simulink model "Inverse_dynamic_Cartesian_aJacobian"  (R2020b)
settings: Solver=VariableStepAuto  StartTime=0.0  StopTime=10.0  RelTol=1e-3
(part 5 of 5)

== matlab function Inverse_dynamic_Cartesian_aJacobian/Controller/MATLAB Function ==
  data: Minimal input size=6; Minimald input; Jd output; Theta input size=6; Thetad input size=6
function Jd = JdAnalytical(Minimal,Minimald,Theta,Thetad)
alpha=Minimal(4);
beta=Minimal(5);
gamma=Minimal(6);
alphad=Minimald(4);
betad=Minimald(5);
gammad=Minimald(6);
t1=Theta(1);
t2=Theta(2);
t3=Theta(3);
t4=Theta(4);
t5=Theta(5);
t6=Theta(6);
td1=Thetad(1);
td2=Thetad(2);
td3=Thetad(3);
td4=Thetad(4);
td5=Thetad(5);
td6=Thetad(6);

Jd = [td2*(408*cos(t2)*sin(t1) - 376*sin(t1)*sin(t2)*sin(t3) + 376*cos(t2)*cos(t3)*sin(t1) + (205*cos(t2)*cos(t3)*cos(t4)*sin(t1))/2 - (205*cos(t2)*sin(t1)*sin(t3)*sin(t4))/2 - (205*cos(t3)*sin(t1)*sin(t2)*sin(t4))/2 - (205*cos(t4)*sin(t1)*sin(t2)*sin(t3))/2 + 94*cos(t2)*cos(t3)*sin(t1)*sin(t4)*sin(t5) + 94*cos(t2)*cos(t4)*sin(t1)*sin(t3)*sin(t5) + 94*cos(t3)*cos(t4)*sin(t1)*sin(t2)*sin(t5) - 94*sin(t1)*sin(t2)*sin(t3)*sin(t4)*sin(t5)) + td1*(408*cos(t1)*sin(t2) - (281*sin(t1))/2 - 94*cos(t5)*sin(t1) + 376*cos(t1)*cos(t2)*sin(t3) + 376*cos(t1)*cos(t3)*sin(t2) + (205*cos(t1)*cos(t2)*cos(t3)*sin(t4))/2 + (205*cos(t1)*cos(t2)*cos(t4)*sin(t3))/2 + (205*cos(t1)*cos(t3)*cos(t4)*sin(t2))/2 - (205*cos(t1)*sin(t2)*sin(t3)*sin(t4))/2 - 94*cos(t1)*cos(t2)*cos(t3)*cos(t4)*sin(t5) + 94*cos(t1)*cos(t2)*sin(t3)*sin(t4)*sin(t5) + 94*cos(t1)*cos(t3)*sin(t2)*sin(t4)*sin(t5) + 94*cos(t1)*cos(t4)*sin(t2)*sin(t3)*sin(t5)) + td4*((205*cos(t2)*cos(t3)*cos(t4)*sin(t1))/2 - (205*cos(t2)*sin(t1)*sin(t3)*sin(t4))/2 - (205*cos(t3)*sin(t1)*sin(t2)*sin(t4))/2 - (205*cos(t4)*sin(t1)*sin(t2)*sin(t3))/2 + 94*cos(t2)*cos(t3)*sin(t1)*sin(t4)*sin(t5) + 94*cos(t2)*cos(t4)*sin(t1)*sin(t3)*sin(t5) + 94*cos(t3)*cos(t4)*sin(t1)*sin(t2)*sin(t5) - 94*sin(t1)*sin(t2)*sin(t3)*sin(t4)*sin(t5)), td1*sin(t1)*((205*cos(t2 + t3 + t4))/2 - 47*cos(t2 + t3 + t4 + t5) + 376*cos(t2 + t3) + 408*cos(t2) + 47*cos(t2 + t3 + t4 - t5)) + td2*cos(t1)*(47*sin(t2 + t3 + t4 - t5) + (205*sin(t2 + t3 + t4))/2 - 47*sin(t2 + t3 + t4 + t5) + 376*sin(t2 + t3) + 408*sin(t2)) + td4*cos(t1)*(47*sin(t2 + t3 + t4 - t5) + (205*sin(t2 + t3 + t4))/2 - 47*sin(t2 + t3 + t4 + t5)), td2*cos(t1)*(47*sin(t2 + t3 + t4 - t5) + (205*sin(t2 + t3 + t4))/2 - 47*sin(t2 + t3 + t4 + t5) + 376*sin(t2 + t3)) + td1*sin(t1)*((205*cos(t2 + t3 + t4))/2 - 47*cos(t2 + t3 + t4 + t5) + 376*cos(t2 + t3) + 47*cos(t2 + t3 + t4 - t5)) + td4*cos(t1)*(47*sin(t2 + t3 + t4 - t5) + (205*sin(t2 + t3 + t4))/2 - 47*sin(t2 + t3 + t4 + t5)), td1*sin(t1)*((205*cos(t2 + t3 + t4))/2 - 47*cos(t2 + t3 + t4 + t5) + 47*cos(t2 + t3 + t4 - t5)) + td2*cos(t1)*(47*sin(t2 + t3 + t4 - t5) + (205*sin(t2 + t3 + t4))/2 - 47*sin(t2 + t3 + t4 + t5)) + td4*cos(t1)*(47*sin(t2 + t3 + t4 - t5) + (205*sin(t2 + t3 + t4))/2 - 47*sin(t2 + t3 + t4 + t5)),                                                                                                                                                                                                                                                                                                                                                                                                                                                                                                        94*td1*cos(t2)*cos(t5)*sin(t1)*sin(t3)*sin(t4) - 94*td2*sin(t2 + t3 + t4)*cos(t1)*cos(t5) - 94*td4*sin(t2 + t3 + t4)*cos(t1)*cos(t5) - 94*td1*cos(t2)*cos(t3)*cos(t4)*cos(t5)*sin(t1) - 94*td1*cos(t1)*sin(t5) + 94*td1*cos(t3)*cos(t5)*sin(t1)*sin(t2)*sin(t4) + 94*td1*cos(t4)*cos(t5)*sin(t1)*sin(t2)*sin(t3),                                                                                                                                                                                                                                                                                                                                                                                                                                                                                                                                                                                                                                                                                                                                                                                                                                                                                                                                                                                                                                                                                                                                                                                                                                                                                                                                             0
td1*((281*cos(t1))/2 + 94*cos(t1)*cos(t5) + 408*sin(t1)*sin(t2) + 376*cos(t2)*sin(t1)*sin(t3) + 376*cos(t3)*sin(t1)*sin(t2) + (205*cos(t2)*cos(t3)*sin(t1)*sin(t4))/2 + (205*cos(t2)*cos(t4)*sin(t1)*sin(t3))/2 + (205*cos(t3)*cos(t4)*sin(t1)*sin(t2))/2 - (205*sin(t1)*sin(t2)*sin(t3)*sin(t4))/2 - 94*cos(t2)*cos(t3)*cos(t4)*sin(t1)*sin(t5) + 94*cos(t2)*sin(t1)*sin(t3)*sin(t4)*sin(t5) + 94*cos(t3)*sin(t1)*sin(t2)*sin(t4)*sin(t5) + 94*cos(t4)*sin(t1)*sin(t2)*sin(t3)*sin(t5)) - td2*(408*cos(t1)*cos(t2) - 376*cos(t1)*sin(t2)*sin(t3) + 376*cos(t1)*cos(t2)*cos(t3) + (205*cos(t1)*cos(t2)*cos(t3)*cos(t4))/2 - (205*cos(t1)*cos(t2)*sin(t3)*sin(t4))/2 - (205*cos(t1)*cos(t3)*sin(t2)*sin(t4))/2 - (205*cos(t1)*cos(t4)*sin(t2)*sin(t3))/2 + 94*cos(t1)*cos(t2)*cos(t3)*sin(t4)*sin(t5) + 94*cos(t1)*cos(t2)*cos(t4)*sin(t3)*sin(t5) + 94*cos(t1)*cos(t3)*cos(t4)*sin(t2)*sin(t5) - 94*cos(t1)*sin(t2)*sin(t3)*sin(t4)*sin(t5)) - td4*((205*cos(t1)*cos(t2)*cos(t3)*cos(t4))/2 - (205*cos(t1)*cos(t2)*sin(t3)*sin(t4))/2 - (205*cos(t1)*cos(t3)*sin(t2)*sin(t4))/2 - (205*cos(t1)*cos(t4)*sin(t2)*sin(t3))/2 + 94*cos(t1)*cos(t2)*cos(t3)*sin(t4)*sin(t5) + 94*cos(t1)*cos(t2)*cos(t4)*sin(t3)*sin(t5) + 94*cos(t1)*cos(t3)*cos(t4)*sin(t2)*sin(t5) - 94*cos(t1)*sin(t2)*sin(t3)*sin(t4)*sin(t5)), td4*sin(t1)*(47*sin(t2 + t3 + t4 - t5) + (205*sin(t2 + t3 + t4))/2 - 47*sin(t2 + t3 + t4 + t5)) - td1*cos(t1)*((205*cos(t2 + t3 + t4))/2 - 47*cos(t2 + t3 + t4 + t5) + 376*cos(t2 + t3) + 408*cos(t2) + 47*cos(t2 + t3 + t4 - t5)) + td2*sin(t1)*(47*sin(t2 + t3 + t4 - t5) + (205*sin(t2 + t3 + t4))/2 - 47*sin(t2 + t3 + t4 + t5) + 376*sin(t2 + t3) + 408*sin(t2)), td4*sin(t1)*(47*sin(t2 + t3 + t4 - t5) + (205*sin(t2 + t3 + t4))/2 - 47*sin(t2 + t3 + t4 + t5)) + td2*sin(t1)*(47*sin(t2 + t3 + t4 - t5) + (205*sin(t2 + t3 + t4))/2 - 47*sin(t2 + t3 + t4 + t5) + 376*sin(t2 + t3)) - td1*cos(t1)*((205*cos(t2 + t3 + t4))/2 - 47*cos(t2 + t3 + t4 + t5) + 376*cos(t2 + t3) + 47*cos(t2 + t3 + t4 - t5)), td2*sin(t1)*(47*sin(t2 + t3 + t4 - t5) + (205*sin(t2 + t3 + t4))/2 - 47*sin(t2 + t3 + t4 + t5)) + td4*sin(t1)*(47*sin(t2 + t3 + t4 - t5) + (205*sin(t2 + t3 + t4))/2 - 47*sin(t2 + t3 + t4 + t5)) - td1*cos(t1)*((205*cos(t2 + t3 + t4))/2 - 47*cos(t2 + t3 + t4 + t5) + 47*cos(t2 + t3 + t4 - t5)),                                                                                                                                                                                                                                                                                                                                                                                                                                                                                                        94*td1*cos(t1)*cos(t2)*cos(t3)*cos(t4)*cos(t5) - 94*td2*sin(t2 + t3 + t4)*cos(t5)*sin(t1) - 94*td4*sin(t2 + t3 + t4)*cos(t5)*sin(t1) - 94*td1*sin(t1)*sin(t5) - 94*td1*cos(t1)*cos(t2)*cos(t5)*sin(t3)*sin(t4) - 94*td1*cos(t1)*cos(t3)*cos(t5)*sin(t2)*sin(t4) - 94*td1*cos(t1)*cos(t4)*cos(t5)*sin(t2)*sin(t3),                                                                                                                                                                                                                                                                                                                                                                                                                                                                                                                                                                                                                                                                                                                                                                                                                                                                                                                                                                                                                                                                                                                                                                                                                                                                                                                                             0
                                                                                                                                                                                                                                                                                                                                                                                                                                                                                                                                                                                                                                                                                                                                                                                                                                                                                                                                                                                                                                                                                                                                                                                                                                                                                                             0,                                                                                                                                                  - td2*((205*cos(t2 + t3 + t4))/2 - 47*cos(t2 + t3 + t4 + t5) + 376*cos(t2 + t3) + 408*cos(t2) + 47*cos(t2 + t3 + t4 - t5)) - td4*((205*cos(t2 + t3 + t4))/2 - 47*cos(t2 + t3 + t4 + t5) + 47*cos(t2 + t3 + t4 - t5)),                                                                                                                                    - td4*((205*cos(t2 + t3 + t4))/2 - 47*cos(t2 + t3 + t4 + t5) + 47*cos(t2 + t3 + t4 - t5)) - td2*((205*cos(t2 + t3 + t4))/2 - 47*cos(t2 + t3 + t4 + t5) + 376*cos(t2 + t3) + 47*cos(t2 + t3 + t4 - t5)),                                                                                                                                                                                                    -((td2 + td4)*(205*cos(t2 + t3 + t4) - 94*cos(t2 + t3 + t4 + t5) + 94*cos(t2 + t3 + t4 - t5)))/2,                                                                                                                                                                                                                                                                                                                                                                                                                                                                                                                                                                                                                                                                                                                                                        47*(td2 + td4)*(cos(t2 + t3 + t4 + t5) + cos(t2 + t3 + t4 - t5)),                                                                                                                                                                                                                                                                                                                                                                                                                                                                                                                                                                                                                                                                                                                                                                                                                                                                                                                                                                                                                                                                                                                                                                                                                                                                                                                                             0
                                                                                                                                                                                                                                                                                                                                                                                                                                                                                                                                                                                                                                                                                                                                                                                                                                                                                                                                                                                                                                                                                                                                                                                                                                                                                                             0,                                                                                         (cos(t1)*(betad*sin(alpha) - alphad*cos(alpha)*cos(beta)*sin(beta)))/(cos(beta)^2 - 1) - (sin(t1)*(betad*cos(alpha) + alphad*cos(beta)*sin(alpha)*sin(beta)))/(cos(beta)^2 - 1) - (td1*cos(alpha)*cos(beta)*cos(t1))/sin(beta) - (td1*cos(beta)*sin(alpha)*sin(t1))/sin(beta),                                                             (cos(t1)*(betad*sin(alpha) - alphad*cos(alpha)*cos(beta)*sin(beta)))/(cos(beta)^2 - 1) - (sin(t1)*(betad*cos(alpha) + alphad*cos(beta)*sin(alpha)*sin(beta)))/(cos(beta)^2 - 1) - (td1*cos(alpha)*cos(beta)*cos(t1))/sin(beta) - (td1*cos(beta)*sin(alpha)*sin(t1))/sin(beta),                       (cos(t1)*(betad*sin(alpha) - alphad*cos(alpha)*cos(beta)*sin(beta)))/(cos(beta)^2 - 1) - (sin(t1)*(betad*cos(alpha) + alphad*cos(beta)*sin(alpha)*sin(beta)))/(cos(beta)^2 - 1) - (td1*cos(alpha)*cos(beta)*cos(t1))/sin(beta) - (td1*cos(beta)*sin(alpha)*sin(t1))/sin(beta), (betad*(sin(alpha) + (cos(beta)^2*sin(alpha))/sin(beta)^2) - (alphad*cos(alpha)*cos(beta))/sin(beta))*(cos(t1 + t2 + t3 + t4)/2 - cos(t2 - t1 + t3 + t4)/2) - td4*sin(t2 + t3 + t4) - td2*sin(t2 + t3 + t4) - (betad*(cos(alpha) + (cos(alpha)*cos(beta)^2)/sin(beta)^2) + (alphad*cos(beta)*sin(alpha))/sin(beta))*(sin(t2 - t1 + t3 + t4)/2 + sin(t1 + t2 + t3 + t4)/2) - (cos(beta)*sin(alpha)*(td2*(sin(t2 - t1 + t3 + t4)/2 - sin(t1 + t2 + t3 + t4)/2) - td1*(sin(t2 - t1 + t3 + t4)/2 + sin(t1 + t2 + t3 + t4)/2) + td4*(sin(t2 - t1 + t3 + t4)/2 - sin(t1 + t2 + t3 + t4)/2)))/sin(beta) + (cos(alpha)*cos(beta)*(td1*(cos(t1 + t2 + t3 + t4)/2 - cos(t2 - t1 + t3 + t4)/2) + td2*(cos(t1 + t2 + t3 + t4)/2 + cos(t2 - t1 + t3 + t4)/2) + td4*(cos(t1 + t2 + t3 + t4)/2 + cos(t2 - t1 + t3 + t4)/2)))/sin(beta), ((betad*cos(alpha) + alphad*cos(beta)*sin(alpha)*sin(beta))*(cos(t1)*cos(t2)*sin(t3)*sin(t4)*sin(t5) - cos(t1)*cos(t2)*cos(t3)*cos(t4)*sin(t5) - cos(t5)*sin(t1) + cos(t1)*cos(t3)*sin(t2)*sin(t4)*sin(t5) + cos(t1)*cos(t4)*sin(t2)*sin(t3)*sin(t5)))/(cos(beta)^2 - 1) - (td4*(sin(t2 + t3 + t4 - t5) - sin(t2 + t3 + t4 + t5)))/2 - (td2*(sin(t2 + t3 + t4 - t5) - sin(t2 + t3 + t4 + t5)))/2 + ((betad*sin(alpha) - alphad*cos(alpha)*cos(beta)*sin(beta))*(cos(t1)*cos(t5) - cos(t2)*cos(t3)*cos(t4)*sin(t1)*sin(t5) + cos(t2)*sin(t1)*sin(t3)*sin(t4)*sin(t5) + cos(t3)*sin(t1)*sin(t2)*sin(t4)*sin(t5) + cos(t4)*sin(t1)*sin(t2)*sin(t3)*sin(t5)))/(cos(beta)^2 - 1) + (cos(beta)*sin(alpha)*(td2*sin(t2 + t3 + t4)*sin(t1)*sin(t5) - td1*cos(t5)*sin(t1) + td4*sin(t2 + t3 + t4)*sin(t1)*sin(t5) - td1*cos(t1)*cos(t2)*cos(t3)*cos(t4)*sin(t5) + td1*cos(t1)*cos(t2)*sin(t3)*sin(t4)*sin(t5) + td1*cos(t1)*cos(t3)*sin(t2)*sin(t4)*sin(t5) + td1*cos(t1)*cos(t4)*sin(t2)*sin(t3)*sin(t5)))/sin(beta) - (cos(alpha)*cos(beta)*(td1*cos(t1)*cos(t5) - td2*sin(t2 + t3 + t4)*cos(t1)*sin(t5) - td4*sin(t2 + t3 + t4)*cos(t1)*sin(t5) - td1*cos(t2)*cos(t3)*cos(t4)*sin(t1)*sin(t5) + td1*cos(t2)*sin(t1)*sin(t3)*sin(t4)*sin(t5) + td1*cos(t3)*sin(t1)*sin(t2)*sin(t4)*sin(t5) + td1*cos(t4)*sin(t1)*sin(t2)*sin(t3)*sin(t5)))/sin(beta)
                                                                                                                                                                                                                                                                                                                                                                                                                                                                                                                                                                                                                                                                                                                                                                                                                                                                                                                                                                                                                                                                                                                                                                                                                                                                                                             0,                                                                                                                                                                                                                                                                                                                                        sin(alpha - t1)*(alphad - td1),                                                                                                                                                                                                                                                                                                            sin(alpha - t1)*(alphad - td1),                                                                                                                                                                                                                                                                      sin(alpha - t1)*(alphad - td1),                                                                                                                                                                                                                                                                                                                                                                                                                                                                             (alphad*sin(alpha - t1 + t2 + t3 + t4))/2 + (alphad*sin(t1 - alpha + t2 + t3 + t4))/2 - (td1*sin(alpha - t1 + t2 + t3 + t4))/2 - (td1*sin(t1 - alpha + t2 + t3 + t4))/2 + (td2*sin(alpha - t1 + t2 + t3 + t4))/2 - (td2*sin(t1 - alpha + t2 + t3 + t4))/2 + (td4*sin(alpha - t1 + t2 + t3 + t4))/2 - (td4*sin(t1 - alpha + t2 + t3 + t4))/2,                                                                                                                                                                                                                                                                                               alphad*sin(alpha)*(cos(t1)*cos(t5) - cos(t2)*cos(t3)*cos(t4)*sin(t1)*sin(t5) + cos(t2)*sin(t1)*sin(t3)*sin(t4)*sin(t5) + cos(t3)*sin(t1)*sin(t2)*sin(t4)*sin(t5) + cos(t4)*sin(t1)*sin(t2)*sin(t3)*sin(t5)) - sin(alpha)*(td1*cos(t1)*cos(t5) - td2*sin(t2 + t3 + t4)*cos(t1)*sin(t5) - td4*sin(t2 + t3 + t4)*cos(t1)*sin(t5) - td1*cos(t2)*cos(t3)*cos(t4)*sin(t1)*sin(t5) + td1*cos(t2)*sin(t1)*sin(t3)*sin(t4)*sin(t5) + td1*cos(t3)*sin(t1)*sin(t2)*sin(t4)*sin(t5) + td1*cos(t4)*sin(t1)*sin(t2)*sin(t3)*sin(t5)) - cos(alpha)*(td2*sin(t2 + t3 + t4)*sin(t1)*sin(t5) - td1*cos(t5)*sin(t1) + td4*sin(t2 + t3 + t4)*sin(t1)*sin(t5) - td1*cos(t1)*cos(t2)*cos(t3)*cos(t4)*sin(t5) + td1*cos(t1)*cos(t2)*sin(t3)*sin(t4)*sin(t5) + td1*cos(t1)*cos(t3)*sin(t2)*sin(t4)*sin(t5) + td1*cos(t1)*cos(t4)*sin(t2)*sin(t3)*sin(t5)) + alphad*cos(alpha)*(cos(t1)*cos(t2)*sin(t3)*sin(t4)*sin(t5) - cos(t1)*cos(t2)*cos(t3)*cos(t4)*sin(t5) - cos(t5)*sin(t1) + cos(t1)*cos(t3)*sin(t2)*sin(t4)*sin(t5) + cos(t1)*cos(t4)*sin(t2)*sin(t3)*sin(t5))
                                                                                                                                                                                                                                                                                                                                                                                                                                                                                                                                                                                                                                                                                                                                                                                                                                                                                                                                                                                                                                                                                                                                                                                                                                                                                                             0,                                                                                                                              -(alphad*cos(alpha)*sin(beta)*cos(t1) + betad*cos(alpha)*cos(beta)*sin(t1) - betad*cos(beta)*sin(alpha)*cos(t1) - td1*cos(alpha)*sin(beta)*cos(t1) + alphad*sin(alpha)*sin(beta)*sin(t1) - td1*sin(alpha)*sin(beta)*sin(t1))/sin(beta)^2,                                                                                                  -(alphad*cos(alpha)*sin(beta)*cos(t1) + betad*cos(alpha)*cos(beta)*sin(t1) - betad*cos(beta)*sin(alpha)*cos(t1) - td1*cos(alpha)*sin(beta)*cos(t1) + alphad*sin(alpha)*sin(beta)*sin(t1) - td1*sin(alpha)*sin(beta)*sin(t1))/sin(beta)^2,                                                            -(alphad*cos(alpha)*sin(beta)*cos(t1) + betad*cos(alpha)*cos(beta)*sin(t1) - betad*cos(beta)*sin(alpha)*cos(t1) - td1*cos(alpha)*sin(beta)*cos(t1) + alphad*sin(alpha)*sin(beta)*sin(t1) - td1*sin(alpha)*sin(beta)*sin(t1))/sin(beta)^2,                                                                                                                           (cos(t1 + t2 + t3 + t4)/2 - cos(t2 - t1 + t3 + t4)/2)*((alphad*cos(alpha))/sin(beta) - (betad*cos(beta)*sin(alpha))/sin(beta)^2) + ((alphad*sin(alpha))/sin(beta) + (betad*cos(alpha)*cos(beta))/sin(beta)^2)*(sin(t2 - t1 + t3 + t4)/2 + sin(t1 + t2 + t3 + t4)/2) - (cos(alpha)*(td1*(cos(t1 + t2 + t3 + t4)/2 - cos(t2 - t1 + t3 + t4)/2) + td2*(cos(t1 + t2 + t3 + t4)/2 + cos(t2 - t1 + t3 + t4)/2) + td4*(cos(t1 + t2 + t3 + t4)/2 + cos(t2 - t1 + t3 + t4)/2)))/sin(beta) + (sin(alpha)*(td2*(sin(t2 - t1 + t3 + t4)/2 - sin(t1 + t2 + t3 + t4)/2) - td1*(sin(t2 - t1 + t3 + t4)/2 + sin(t1 + t2 + t3 + t4)/2) + td4*(sin(t2 - t1 + t3 + t4)/2 - sin(t1 + t2 + t3 + t4)/2)))/sin(beta),                                                                                                                                                         ((betad*cos(alpha)*cos(beta) + alphad*sin(alpha)*sin(beta))*(cos(t1)*cos(t2)*sin(t3)*sin(t4)*sin(t5) - cos(t1)*cos(t2)*cos(t3)*cos(t4)*sin(t5) - cos(t5)*sin(t1) + cos(t1)*cos(t3)*sin(t2)*sin(t4)*sin(t5) + cos(t1)*cos(t4)*sin(t2)*sin(t3)*sin(t5)))/sin(beta)^2 - ((alphad*cos(alpha)*sin(beta) - betad*cos(beta)*sin(alpha))*(cos(t1)*cos(t5) - cos(t2)*cos(t3)*cos(t4)*sin(t1)*sin(t5) + cos(t2)*sin(t1)*sin(t3)*sin(t4)*sin(t5) + cos(t3)*sin(t1)*sin(t2)*sin(t4)*sin(t5) + cos(t4)*sin(t1)*sin(t2)*sin(t3)*sin(t5)))/sin(beta)^2 - (sin(alpha)*(td2*sin(t2 + t3 + t4)*sin(t1)*sin(t5) - td1*cos(t5)*sin(t1) + td4*sin(t2 + t3 + t4)*sin(t1)*sin(t5) - td1*cos(t1)*cos(t2)*cos(t3)*cos(t4)*sin(t5) + td1*cos(t1)*cos(t2)*sin(t3)*sin(t4)*sin(t5) + td1*cos(t1)*cos(t3)*sin(t2)*sin(t4)*sin(t5) + td1*cos(t1)*cos(t4)*sin(t2)*sin(t3)*sin(t5)))/sin(beta) + (cos(alpha)*(td1*cos(t1)*cos(t5) - td2*sin(t2 + t3 + t4)*cos(t1)*sin(t5) - td4*sin(t2 + t3 + t4)*cos(t1)*sin(t5) - td1*cos(t2)*cos(t3)*cos(t4)*sin(t1)*sin(t5) + td1*cos(t2)*sin(t1)*sin(t3)*sin(t4)*sin(t5) + td1*cos(t3)*sin(t1)*sin(t2)*sin(t4)*sin(t5) + td1*cos(t4)*sin(t1)*sin(t2)*sin(t3)*sin(t5)))/sin(beta)];

== matlab function Inverse_dynamic_Cartesian_aJacobian/Controller/MATLAB Function1 ==
  data: JA input; Jinv output
function Jinv = JacAnalyticalInv(JA)

Jinv=JA^(-1);

== matlab function Inverse_dynamic_Cartesian_aJacobian/Controller/Gain Calculator ==
  data: Ts input; DesiredInputdd input; xdd output; Errord input; Error input
function xdd = GainCalc(Ts,DesiredInputdd,Errord,Error)
ZETTA=1;

OMEGA=4/ZETTA/Ts;
Kp=diag(OMEGA^2*ones(6,1));
Kd=diag(2*ZETTA*OMEGA*ones(6,1));

xdd=DesiredInputdd+Kd*Errord+Kp*Error;
